simulink model "Final_Project"  (R2023b)
settings: Solver=VariableStepAuto  StartTime=0.0  StopTime=10  RelTol=1e-3
values from neighbouring files (symbols this model uses):
  c = 0.8    [CORRECTED_HW_13_4.m]    (also in CORRECTED_HW_14_3.m; Final_Project_State_Space.m = 10; Homework13_4.m; twomassdata.m)
  c2 = 10    [Final_Project_State_Space.m]    (also in untitled.m = 100; untitled2.m = 100)
  k1 = 18    [CORRECTED_HW_13_4.m]    (also in CORRECTED_HW_14_3.m; Final_Project_State_Space.m = 13650; Homework13_4.m; twomassdata.m)
  k2 = 21    [CORRECTED_HW_13_4.m]    (also in CORRECTED_HW_14_3.m; Final_Project_State_Space.m = 13650; Homework13_4.m; twomassdata.m)
  m1 = 1    [CORRECTED_HW_13_4.m]    (also in CORRECTED_HW_14_3.m; Final_Project_State_Space.m = 3000; Homework13_4.m; twomassdata.m)
  m2 = 1.4    [CORRECTED_HW_13_4.m]    (also in CORRECTED_HW_14_3.m; Final_Project_State_Space.m = 12000; Homework13_4.m; twomassdata.m)
settings Model: Creator=Todd McKenzie  LastModifiedBy=Todd McKenzie

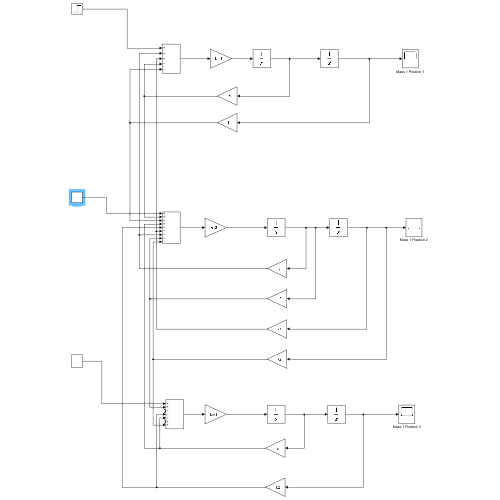
[thumbnail: Simulink's stored preview of the top-level diagram]
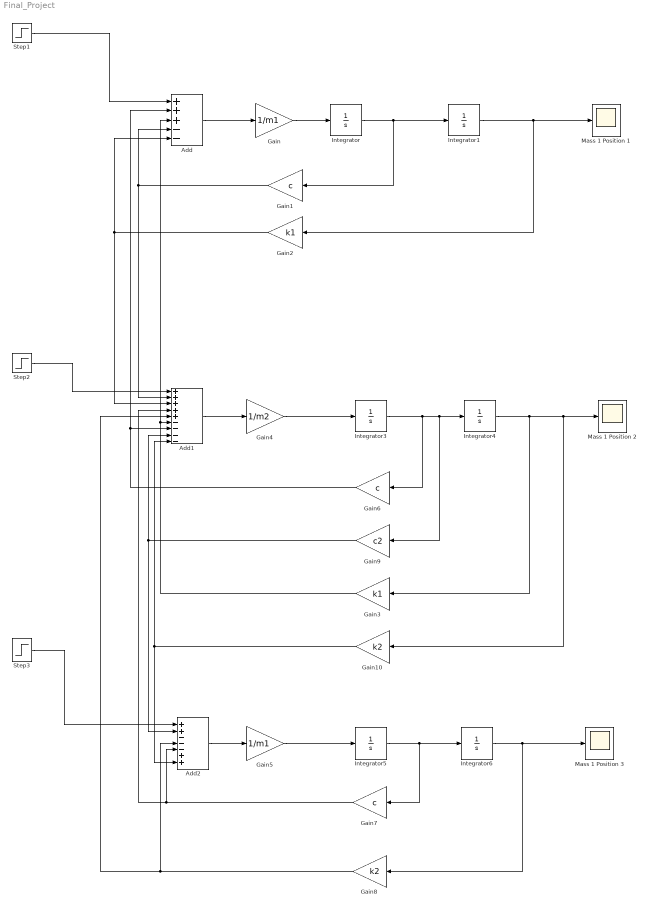
== system Final_Project ==
  Add : Sum  Inputs=+++--
  Add1 : Sum  Inputs=+++++----
  Add2 : Sum  Inputs=++---++
  Gain : Gain  Gain=1/m1
  Gain1 : Gain  Gain=c
  Gain10 : Gain  Gain=k2
  Gain2 : Gain  Gain=k1
  Gain3 : Gain  Gain=k1
  Gain4 : Gain  Gain=1/m2
  Gain5 : Gain  Gain=1/m1
  Gain6 : Gain  Gain=c
  Gain7 : Gain  Gain=c
  Gain8 : Gain  Gain=k2
  Gain9 : Gain  Gain=c2
  Integrator{,1,3..6} (6 alike) : Integrator
  Mass 1 Position 1 : Scope
  Mass 1 Position 2 : Scope
  Mass 1 Position 3 : Scope
  Step1 : Step  Time=0  After=0  SampleTime=0
  Step2 : Step  Time=0  SampleTime=0
  Step3 : Step  Time=0  After=0  SampleTime=0
  wires:
  Add/1 -> Gain/1
  Gain/1 -> Integrator/1
  Integrator/1 -> Integrator1/1, Gain1/1
  Integrator1/1 -> Mass 1 Position 1/1, Gain2/1
  Step3/1 -> Add2/1
  Add1/1 -> Gain4/1
  Add2/1 -> Gain5/1
  Gain4/1 -> Integrator3/1
  Integrator3/1 -> Gain6/1, Gain9/1, Integrator4/1
  Gain5/1 -> Integrator5/1
  Integrator5/1 -> Gain7/1, Integrator6/1
  Integrator6/1 -> Mass 1 Position 3/1, Gain8/1
  Step1/1 -> Add/1
  Gain1/1 -> Add/4, Add1/2
  Gain2/1 -> Add/5, Add1/3
  Gain9/1 -> Add2/2, Add1/8
  Integrator4/1 -> Gain3/1, Gain10/1, Mass 1 Position 2/1
  Gain6/1 -> Add/2, Add1/7
  Gain3/1 -> Add1/6, Add/3
  Gain10/1 -> Add2/7, Add1/9
  Gain7/1 -> Add2/5, Add1/4
  Gain8/1 -> Add2/4, Add1/5
  Step2/1 -> Add1/1
